simulink model "globalSystem"  (R2014b)
settings: Solver=ode45  StartTime=0.0  StopTime=10.0  RelTol=1e-3
settings Model: Creator=Adrien  LastModifiedBy=Adrien

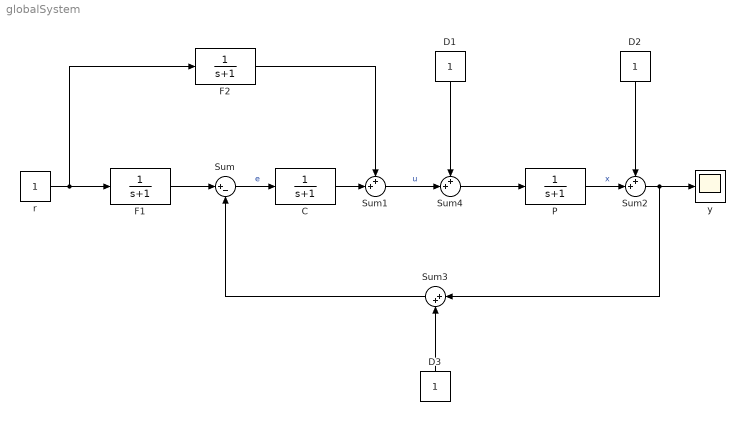
== system globalSystem ==
  C : TransferFcn  Denominator=[1 1]
  D1 : Constant
  D2 : Constant
  D3 : Constant
  F1 : TransferFcn  Denominator=[1 1]
  F2 : TransferFcn  Denominator=[1 1]
  P : TransferFcn  Denominator=[1 1]
  Sum : Sum  Inputs=|+-
  Sum1 : Sum  Inputs=++|
  Sum2 : Sum  Inputs=++|
  Sum3 : Sum  Inputs=|++
  Sum4 : Sum  Inputs=++|
  r : Constant
  y : Scope
  wires:
  r/1 -> F2/1, F1/1
  F1/1 -> Sum/1
  Sum/1 -> C/1  "e"
  C/1 -> Sum1/2
  P/1 -> Sum2/2  "x"
  F2/1 -> Sum1/1
  Sum1/1 -> Sum4/2  "u"
  Sum4/1 -> P/1
  D1/1 -> Sum4/1
  D2/1 -> Sum2/1
  D3/1 -> Sum3/2
  Sum2/1 -> y/1, Sum3/1
  Sum3/1 -> Sum/2
